simulink model "SyncGenNoLib"  (R2013a)
settings: Solver=ode45  StartTime=5  StopTime=10  FixedStep=10^-3  MaxStep=10^-2  RelTol=1e-2
undefined symbols (not defined in the file): D_p, J, L_f, L_s, M_f, R_f, R_l, R_s, T_m, V_f
libraries: powerlib x22, SyncGenLib x2, powerlib_meascontrol x1
settings Model: Creator=Elad  LastModifiedBy=USER
settings DataIOCC: SignalLoggingSaveFormat=ModelDataLogs
settings DebuggingCC: MultiTaskDSMMsg=warning  MultiTaskCondExecSysMsg=none  StateNameClashWarn=none  StrictBusMsg=None
settings RTWCC: IncludeERTFirstTime=on

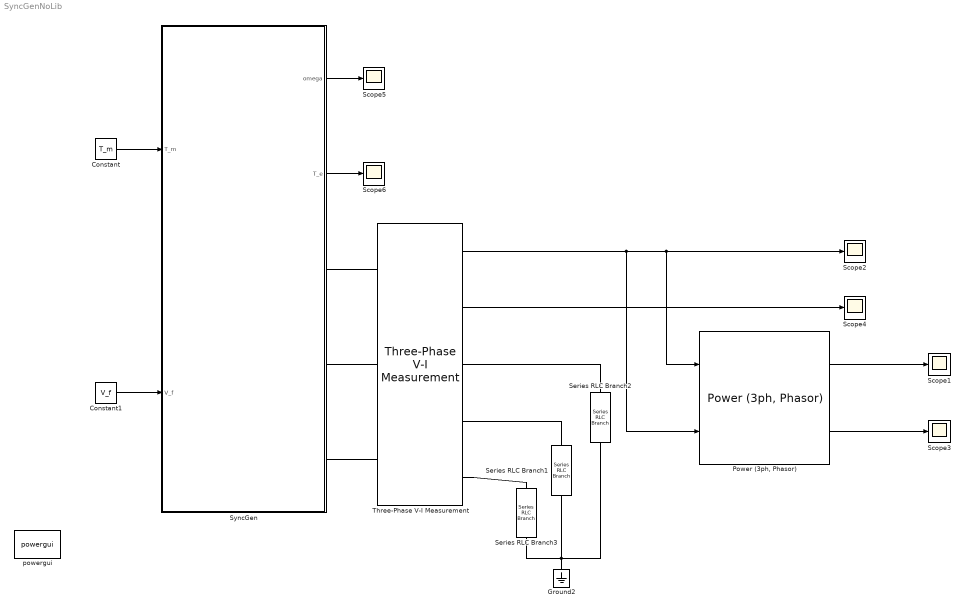
== system SyncGenNoLib ==
  Constant : Constant  Value=T_m
  Constant1 : Constant  Value=V_f
  Ground2 : powerlib/Elements/Ground  LConnTagsString=a
  "Power (3ph, Phasor)" : powerlib_meascontrol/Measurements/Power (3ph, Phasor)
  Scope{1..6} (6 alike) : Scope
      Scope1 settings: TimeRange=5  YMin=720000  YMax=757500
      Scope2 settings: TimeRange=5  YMin=-55  YMax=55  SaveName=ScopeData2
      Scope3 settings: TimeRange=5  YMin=-225  YMax=225  SaveName=ScopeData3
      Scope4 settings: TimeRange=5  YMin=-0.011  YMax=0.011  SaveName=ScopeData4
      Scope5 settings: TimeRange=5  YMin=465.118  YMax=465.13  SaveName=ScopeData5
      Scope6 settings: TimeRange=5  YMin=-7.1  YMax=-6.89  SaveName=ScopeData6
  Series RLC Branch1 : powerlib/Elements/Series RLC Branch  LConnTagsString=__new0  RConnTagsString=__new0  BranchType=R  Resistance=R_l  Inductance=1e-3  SetiL0=off  InitialCurrent=0  Capacitance=1e-6  Setx0=off  InitialVoltage=0  Measurements=None
  Series RLC Branch2 : powerlib/Elements/Series RLC Branch  LConnTagsString=__new0  RConnTagsString=__new0  BranchType=R  Resistance=R_l  Inductance=1e-3  SetiL0=off  InitialCurrent=0  Capacitance=1e-6  Setx0=off  InitialVoltage=0  Measurements=None
  Series RLC Branch3 : powerlib/Elements/Series RLC Branch  LConnTagsString=__new0  RConnTagsString=__new0  BranchType=R  Resistance=R_l  Inductance=1e-3  SetiL0=off  InitialCurrent=0  Capacitance=1e-6  Setx0=off  InitialVoltage=0  Measurements=None
  SyncGen : Subsystem
  Three-Phase V-I Measurement : powerlib/Measurements/Three-Phase V-I Measurement  VoltageMeasurement=phase-to-ground  SetLabelV=off  LabelV=Vabc  Vpu=off  VpuLL=off  CurrentMeasurement=yes  SetLabelI=off  LabelI=Iabc  Ipu=off  Pbase=100e6  Vbase=500e3  OutputType=Complex  PhasorSimulation=off  PSBequivalent=0
  powergui : powerlib/powergui  Priority=1  SimulationMode=Continuous  SolverType=Tustin  SampleTime=50e-6  frequency=60  SPID=off  DisableSnubberDevices=off  DisableRonSwitches=off  DisableVfSwitches=off  SwTol=0  Interpol=off  DisplayEquations=off  frequencyindice=0  Pbase=100e6  ErrMax=1e-4  Iterations=50  UnitsV=kV  UnitsW=MW  FunctionMessages=off  echomessages=off  HookPort=off  EnableUseOfTLC=off  x0status=blocks  RestoreLinks=warning  ResistiveCurrentMeasurement=off  Frange=[0:2:500]  Ylog=off  Xlog=on  ShowGrid=off  save=off  variable=ZData  ZoomFFT=off  StartTime=0.0  cycles=1  DisplayStyle=1  fundamental=60  FreqAxis=off  MaxFrequency=1000  frequencyindicesteady=1  RmsSteady=1  display=off  Ts=0  methode=off
  wires:
  Constant/1 -> SyncGen/1(T_m)
  Constant1/1 -> SyncGen/2(V_f)
  "Power (3ph, Phasor)"/1 -> Scope1/1
  "Power (3ph, Phasor)"/2 -> Scope3/1
  Three-Phase V-I Measurement/1 -> "Power (3ph, Phasor)"/2, "Power (3ph, Phasor)"/1, Scope2/1
  Three-Phase V-I Measurement/2 -> Scope4/1
  SyncGen/1(omega) -> Scope5/1
  SyncGen/2(T_e) -> Scope6/1
  connections:
  SyncGen/RConn2 -- Three-Phase V-I Measurement/LConn2
  SyncGen/RConn1 -- Three-Phase V-I Measurement/LConn1
  Three-Phase V-I Measurement/RConn3 -- Series RLC Branch3/LConn1
  SyncGen/RConn3 -- Three-Phase V-I Measurement/LConn3
  Three-Phase V-I Measurement/RConn2 -- Series RLC Branch1/LConn1
  Three-Phase V-I Measurement/RConn1 -- Series RLC Branch2/LConn1
  Ground2/LConn1 -- Series RLC Branch2/RConn1 -- Series RLC Branch1/RConn1 -- Series RLC Branch3/RConn1

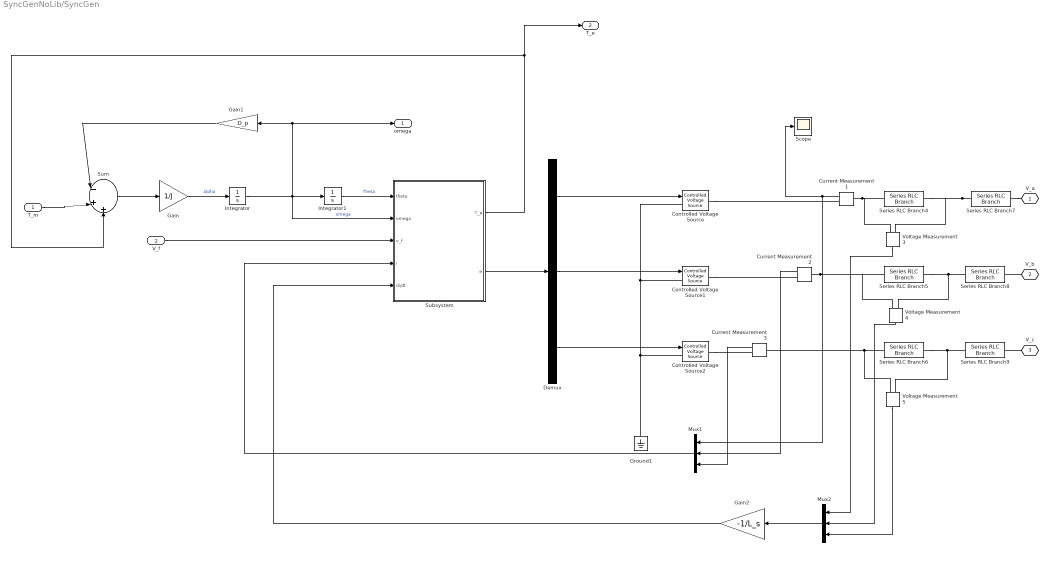
== system SyncGenNoLib/SyncGen ==
  T_m : Inport
  V_f : Inport  Port=2
  Controlled Voltage Source : powerlib/Electrical Sources/Controlled Voltage Source  Initialize=off  Source_Type=AC  Amplitude=0  Phase=0  Frequency=0  Measurements=None
  Controlled Voltage Source1 : powerlib/Electrical Sources/Controlled Voltage Source  Initialize=off  Source_Type=AC  Amplitude=0  Phase=0  Frequency=0  Measurements=None
  Controlled Voltage Source2 : powerlib/Electrical Sources/Controlled Voltage Source  Initialize=off  Source_Type=AC  Amplitude=0  Phase=0  Frequency=0  Measurements=None
  Current Measurement1 : powerlib/Measurements/Current Measurement  PhasorSimulation=off  OutputType=Complex  PSBequivalent=0
  Current Measurement2 : powerlib/Measurements/Current Measurement  PhasorSimulation=off  OutputType=Complex  PSBequivalent=0
  Current Measurement3 : powerlib/Measurements/Current Measurement  PhasorSimulation=off  OutputType=Complex  PSBequivalent=0
  Demux : Demux  Outputs=3
  Gain : Gain  Gain=1/J
  Gain1 : Gain  Gain=D_p
  Gain2 : Gain  Gain=-1/L_s
  Ground1 : powerlib/Elements/Ground  LConnTagsString=a
  Integrator : Integrator
  Integrator1 : Integrator
  Mux1 : Mux  Inputs=3
  Mux2 : Mux  Inputs=3
  Scope : Scope
      settings: YMin=-1  YMax=1
  Series RLC Branch4 : powerlib/Elements/Series RLC Branch  LConnTagsString=__new0  RConnTagsString=__new0  BranchType=L  Resistance=R_s  Inductance=L_s  SetiL0=off  InitialCurrent=0  Capacitance=1e-6  Setx0=off  InitialVoltage=0  Measurements=None
  Series RLC Branch5 : powerlib/Elements/Series RLC Branch  LConnTagsString=__new0  RConnTagsString=__new0  BranchType=L  Resistance=R_s  Inductance=L_s  SetiL0=off  InitialCurrent=0  Capacitance=1e-6  Setx0=off  InitialVoltage=0  Measurements=None
  Series RLC Branch6 : powerlib/Elements/Series RLC Branch  LConnTagsString=__new0  RConnTagsString=__new0  BranchType=L  Resistance=R_s  Inductance=L_s  SetiL0=off  InitialCurrent=0  Capacitance=1e-6  Setx0=off  InitialVoltage=0  Measurements=None
  Series RLC Branch7 : powerlib/Elements/Series RLC Branch  LConnTagsString=__new0  RConnTagsString=__new0  BranchType=R  Resistance=R_s  Inductance=L_s  SetiL0=off  InitialCurrent=0  Capacitance=1e-6  Setx0=off  InitialVoltage=0  Measurements=None
  Series RLC Branch8 : powerlib/Elements/Series RLC Branch  LConnTagsString=__new0  RConnTagsString=__new0  BranchType=R  Resistance=R_s  Inductance=L_s  SetiL0=off  InitialCurrent=0  Capacitance=1e-6  Setx0=off  InitialVoltage=0  Measurements=None
  Series RLC Branch9 : powerlib/Elements/Series RLC Branch  LConnTagsString=__new0  RConnTagsString=__new0  BranchType=R  Resistance=R_s  Inductance=L_s  SetiL0=off  InitialCurrent=0  Capacitance=1e-6  Setx0=off  InitialVoltage=0  Measurements=None
  Subsystem : Subsystem
  Sum : Sum  Inputs=|-++
  Voltage Measurement3 : powerlib/Measurements/Voltage Measurement  PhasorSimulation=off  OutputType=Complex  PSBequivalent=0
  Voltage Measurement4 : powerlib/Measurements/Voltage Measurement  PhasorSimulation=off  OutputType=Complex  PSBequivalent=0
  Voltage Measurement5 : powerlib/Measurements/Voltage Measurement  PhasorSimulation=off  OutputType=Complex  PSBequivalent=0
  V_a : PMIOPort  Tag=PMCPort  Port=1  Side=Right
  V_b : PMIOPort  Tag=PMCPort  Port=2  Side=Right
  V_c : PMIOPort  Tag=PMCPort  Port=3  Side=Right
  omega : Outport
  T_e : Outport  Port=2
  wires:
  Sum/1 -> Gain/1
  Gain/1 -> Integrator/1  "alpha"
  Integrator/1 -> Subsystem/2(omega), omega/1, Gain1/1, Integrator1/1  "omega"
  Gain1/1 -> Sum/1
  T_m/1 -> Sum/2
  Integrator1/1 -> Subsystem/1("theta ")  "Theta"
  Demux/1 -> Controlled Voltage Source/1
  Demux/2 -> Controlled Voltage Source1/1
  Demux/3 -> Controlled Voltage Source2/1
  Subsystem/1("T_e ") -> T_e/1, Sum/3
  Current Measurement1/1 -> Scope/1, Mux1/1
  Current Measurement2/1 -> Mux1/2
  Current Measurement3/1 -> Mux1/3
  Mux1/1 -> Subsystem/4(i)
  Subsystem/2(e) -> Demux/1
  Voltage Measurement3/1 -> Mux2/1
  Voltage Measurement4/1 -> Mux2/2
  Voltage Measurement5/1 -> Mux2/3
  Mux2/1 -> Gain2/1
  Gain2/1 -> Subsystem/5(di/dt)
  V_f/1 -> Subsystem/3(v_f)
  connections:
  Ground1/LConn1 -- Controlled Voltage Source2/LConn1 -- Controlled Voltage Source/LConn1 -- Controlled Voltage Source1/LConn1
  Current Measurement1/LConn1 -- Series RLC Branch4/LConn1 -- Voltage Measurement3/LConn1
  Current Measurement2/LConn1 -- Voltage Measurement4/LConn1 -- Series RLC Branch5/LConn1
  Voltage Measurement5/LConn1 -- Current Measurement3/LConn1 -- Series RLC Branch6/LConn1
  Series RLC Branch7/LConn1 -- Voltage Measurement3/LConn2 -- Series RLC Branch4/RConn1
  Voltage Measurement4/LConn2 -- Series RLC Branch8/LConn1 -- Series RLC Branch5/RConn1
  Voltage Measurement5/LConn2 -- Series RLC Branch9/LConn1 -- Series RLC Branch6/RConn1
  Controlled Voltage Source/RConn1 -- Current Measurement1/RConn1
  Controlled Voltage Source1/RConn1 -- Current Measurement2/RConn1
  Controlled Voltage Source2/RConn1 -- Current Measurement3/RConn1
  Series RLC Branch7/RConn1 -- V_a/RConn1
  V_c/RConn1 -- Series RLC Branch9/RConn1
  V_b/RConn1 -- Series RLC Branch8/RConn1

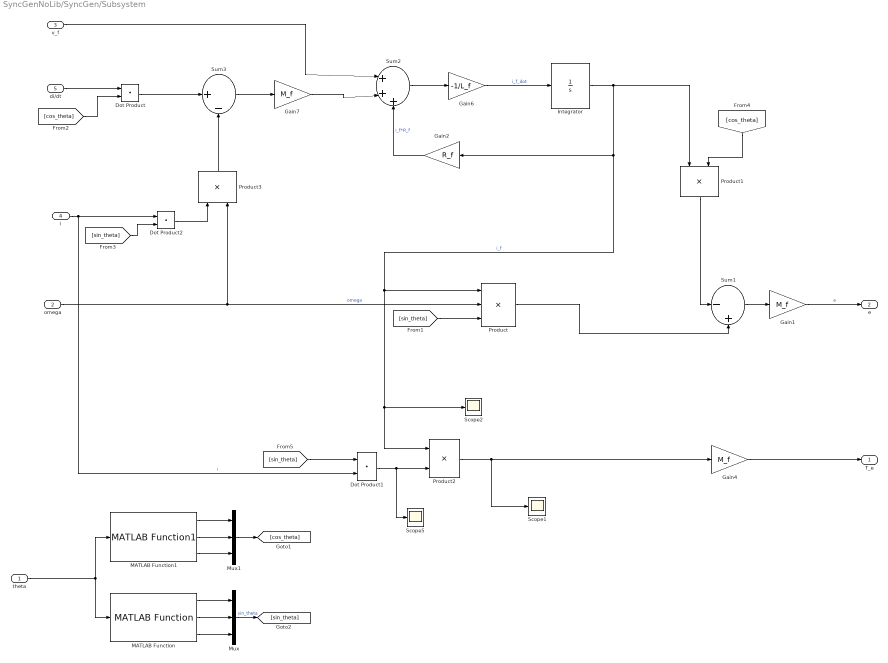
== system SyncGenNoLib/SyncGen/Subsystem ==
  "theta " : Inport  OutDataTypeStr=double
  omega : Inport  Port=2
  v_f : Inport  Port=3
  i : Inport  Port=4
  di/dt : Inport  Port=5
  Dot Product : DotProduct  InputSameDT=on  OutDataTypeStr=Inherit: Inherit via internal rule
  Dot Product1 : DotProduct  InputSameDT=on  OutDataTypeStr=Inherit: Inherit via internal rule
  Dot Product2 : DotProduct  InputSameDT=on  OutDataTypeStr=Inherit: Inherit via internal rule
  Gain1 : Gain  Gain=M_f
  Gain2 : Gain  Gain=R_f
  Gain4 : Gain  Gain=M_f
  Gain6 : Gain  Gain=-1/L_f
  Gain7 : Gain  Gain=M_f
  Integrator : Integrator
  MATLAB Function : SyncGenLib/SyncGen /Subsystem/MATLAB Function
  MATLAB Function1 : SyncGenLib/SyncGen /Subsystem/MATLAB Function1
  Mux : Mux  Inputs=3
  Mux1 : Mux  Inputs=3
  Product : Product  Inputs=3
  Product1 : Product
  Product2 : Product
  Product3 : Product
  Scope1 : Scope
      settings: TimeRange=5  YMin=-55  YMax=55  SaveName=ScopeData8
  Scope2 : Scope
      settings: TimeRange=5  YMin=-55  YMax=55  SaveName=ScopeData9
  Scope5 : Scope
      settings: TimeRange=5  YMin=-55  YMax=55  SaveName=ScopeData7
  Sum1 : Sum  Inputs=|-+
  Sum2 : Sum  Inputs=|+++
  Sum3 : Sum  Inputs=|+-
  "T_e " : Outport
  e : Outport  Port=2
  wires:
  Gain1/1 -> e/1  "e"
  MATLAB Function/1 -> Mux/1
  MATLAB Function/2 -> Mux/2
  MATLAB Function/3 -> Mux/3
  Integrator/1 -> Scope2/1, Product2/1, Product/1, Gain2/1, Product1/1  "i_f"
  MATLAB Function1/1 -> Mux1/1
  MATLAB Function1/2 -> Mux1/2
  MATLAB Function1/3 -> Mux1/3
  Dot Product/1 -> Sum3/1
  i/1 -> Dot Product2/1, Dot Product1/2  "i"
  "theta "/1 -> MATLAB Function/1, MATLAB Function1/1
  omega/1 -> Product3/2, Product/2  "omega"
  Product2/1 -> Scope1/1, Gain4/1
  Sum3/1 -> Gain7/1
  Dot Product2/1 -> Product3/1
  Product3/1 -> Sum3/2
  di/dt/1 -> Dot Product/1
  v_f/1 -> Sum2/1
  Mux1/1 -> [cos_theta]
  Mux/1 -> [sin_theta]  "sin_theta"
  [sin_theta] -> Product/3
  [cos_theta] -> Dot Product/2
  [sin_theta] -> Dot Product2/2
  Gain7/1 -> Sum2/2
  Gain2/1 -> Sum2/3  "i_f*R_f"
  Sum2/1 -> Gain6/1
  Gain6/1 -> Integrator/1  "i_f_dot"
  Product/1 -> Sum1/2
  Product1/1 -> Sum1/1
  [cos_theta] -> Product1/2
  Sum1/1 -> Gain1/1
  [sin_theta] -> Dot Product1/1
  Gain4/1 -> "T_e "/1
  Dot Product1/1 -> Scope5/1, Product2/2
